simulink model "test_AM01"  (R2018b)
settings: Solver=FixedStepAuto  StartTime=0.0  StopTime=T  FixedStep=dt  RelTol=1e-3
undefined symbols (not defined in the file): dt
settings Model: Creator=39926  LastModifiedBy=39926

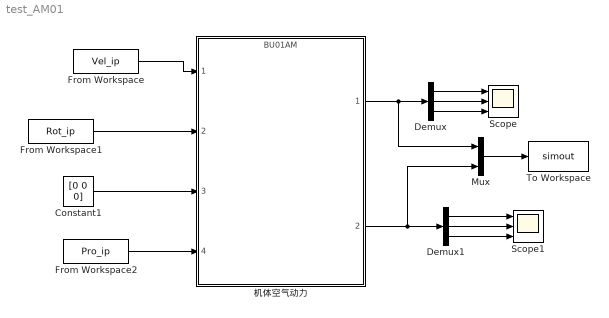
== system test_AM01 ==
  Constant1 : Constant  Value=[0 0 0]  SampleTime=0
  Demux : Demux  Outputs=3
  Demux1 : Demux  Outputs=3
  From Workspace : FromWorkspace  VariableName=Vel_ip  SampleTime=dt
  From Workspace1 : FromWorkspace  VariableName=Rot_ip  SampleTime=dt
  From Workspace2 : FromWorkspace  VariableName=Pro_ip  SampleTime=dt
  Mux : Mux  Inputs=2
  Scope : Scope  NumInputPorts=3
  Scope1 : Scope  NumInputPorts=3
  To Workspace : ToWorkspace  VariableName=simout  SaveFormat=Timeseries  SampleTime=-1
  机体空气动力 : ModelReference  ModelNameDialog=BU01AM.slx  SimulationMode=Normal  ModelReferenceVersion=1.55
  wires:
  From Workspace/1 -> 机体空气动力/1
  From Workspace1/1 -> 机体空气动力/2
  Constant1/1 -> 机体空气动力/3
  From Workspace2/1 -> 机体空气动力/4
  机体空气动力/1 -> Mux/1, Demux/1
  机体空气动力/2 -> Mux/2, Demux1/1
  Demux/1 -> Scope/1
  Demux/2 -> Scope/2
  Demux/3 -> Scope/3
  Demux1/1 -> Scope1/1
  Demux1/2 -> Scope1/2
  Demux1/3 -> Scope1/3
  Mux/1 -> To Workspace/1
